simulink library "singleTether_cl"  (R2018b)
settings: Solver=VariableStepAuto  StartTime=0.0  StopTime=10.0  RelTol=1e-3
values from neighbouring files (symbols this model uses):
  ini_Ri_o = Ri_o    [singleTether_ts.m]
  ini_Vi_o = zeros(size(Vi_o))    [singleTether_ts.m]
  m_i = 2    [singleTether_ts.m]
  N = 20    [singleTether_ts.m]
libraries: tetherBuoyancyAndWeight_ul x1, tetherDragForce_ul x1, tetherInternalForces_ul x1
settings Model: Creator=asiddiq2  LastModifiedBy=asiddiq2

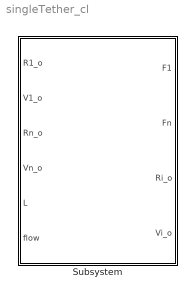
== system singleTether_cl ==
  Subsystem : Subsystem  mask{N=N, dia_t=0, E=0, rho_tether=0, Cd=0, zeta=0, rho_density=0, mass=0, ini_Rn_o=0, ini_R1_o=0}
      mask prompts: N "Number of nodes (N>=2)"; dia_t "Tether diameter (m)"; E "Tether youngs modulus (N/m^2)"; rho_tether "Tether density (kg/m^3)"; Cd "Tether drag coefficient"; zeta "Damping ratio"; rho_density "Fluid density"; mass "Vehicle mass"; ini_Rn_o "Initial vehicle attachment position vector"; ini_R1_o "Initial ground attachment position vector"
      mask DialogControl Container2 Prompt: Tether properties

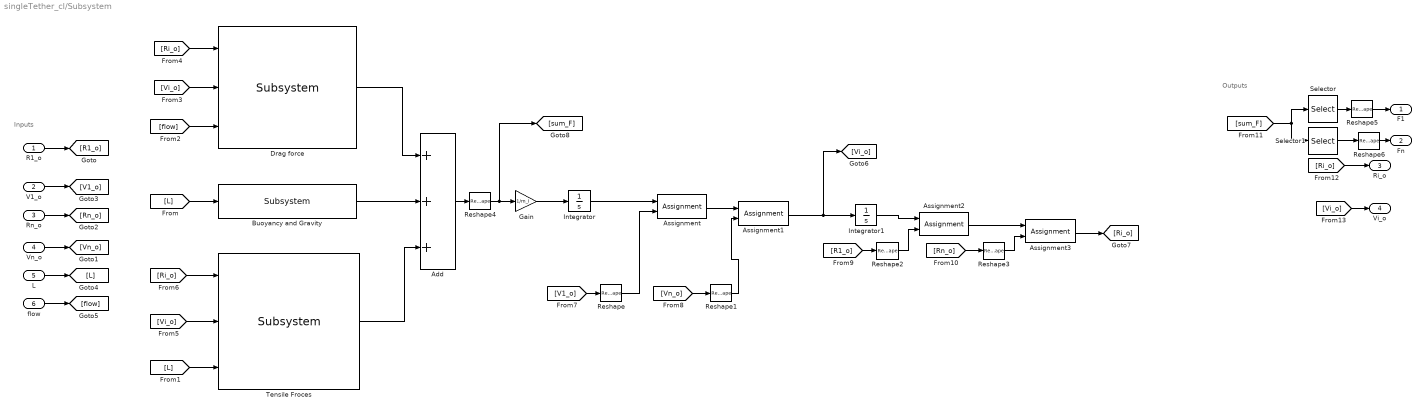
== system singleTether_cl/Subsystem ==
  note: Outputs
  note: Inputs
  R1_o : Inport
  V1_o : Inport  Port=2
  Rn_o : Inport  Port=3
  Vn_o : Inport  Port=4
  L : Inport  Port=5
  flow : Inport  Port=6
  Add : Sum  Inputs=+++
  Assignment : Assignment  NumberOfDimensions=2  DiagnosticForDimensions=Warning  IndexOptions=Index vector (dialog),Assign all  Indices=1,[1 2 3]  OutputSizes=1,1
  Assignment1 : Assignment  NumberOfDimensions=2  DiagnosticForDimensions=Warning  IndexOptions=Index vector (dialog),Assign all  Indices=N,[1 2 3]  OutputSizes=1,1
  Assignment2 : Assignment  NumberOfDimensions=2  DiagnosticForDimensions=Warning  IndexOptions=Index vector (dialog),Assign all  Indices=1,[1 2 3]  OutputSizes=1,1
  Assignment3 : Assignment  NumberOfDimensions=2  DiagnosticForDimensions=Warning  IndexOptions=Index vector (dialog),Assign all  Indices=N,[1 2 3]  OutputSizes=1,1
  Buoyancy and Gravity : tetherBuoyancyAndWeight_ul/Subsystem  N=N  dia_t=dia_t  rho_fluid=rho_fluid  rho_tether=rho_tether  g=9.81
  Drag force : tetherDragForce_ul/Subsystem  Cd=Cd  rho_fluid=rho_fluid  dia_t=dia_t
  Gain : Gain  Gain=1/m_i
  Integrator : Integrator  InitialCondition=ini_Vi_o
  Integrator1 : Integrator  InitialCondition=ini_Ri_o
  Reshape{,1..3} (4 alike) : Reshape  OutputDimensionality=Row vector (2-D)
  Reshape4 : Reshape  OutputDimensionality=Customize  OutputDimensions=[N,3]
  Reshape5 : Reshape  OutputDimensionality=Column vector (2-D)
  Reshape6 : Reshape  OutputDimensionality=Column vector (2-D)
  Selector : Selector  NumberOfDimensions=2  InputPortWidth=3  IndexOptions=Index vector (dialog),Select all  Indices=[1],1  OutputSizes=1,1
  Selector1 : Selector  NumberOfDimensions=2  InputPortWidth=3  IndexOptions=Index vector (dialog),Select all  Indices=[N],1  OutputSizes=1,1
  Tensile Froces : tetherInternalForces_ul/Subsystem  N=N  E=E  dia_t=dia_t  mass=mass  zeta=zeta
  F1 : Outport
  Fn : Outport  Port=2
  Ri_o : Outport  Port=3
  Vi_o : Outport  Port=4
  wires:
  R1_o/1 -> [R1_o]
  V1_o/1 -> [V1_o]
  Rn_o/1 -> [Rn_o]
  Vn_o/1 -> [Vn_o]
  L/1 -> [L]
  flow/1 -> [flow]
  [L] -> Buoyancy and Gravity/1
  [L] -> Tensile Froces/3
  [flow] -> Drag force/3
  Buoyancy and Gravity/1 -> Add/2
  Drag force/1 -> Add/1
  Tensile Froces/1 -> Add/3
  Gain/1 -> Integrator/1
  Integrator/1 -> Assignment/1
  [Vi_o] -> Drag force/2
  [Ri_o] -> Drag force/1
  [Vi_o] -> Tensile Froces/2
  [Ri_o] -> Tensile Froces/1
  [V1_o] -> Reshape/1
  Reshape/1 -> Assignment/2
  Assignment/1 -> Assignment1/1
  [Vn_o] -> Reshape1/1
  Reshape1/1 -> Assignment1/2
  Assignment1/1 -> [Vi_o], Integrator1/1
  [R1_o] -> Reshape2/1
  [Rn_o] -> Reshape3/1
  Reshape2/1 -> Assignment2/2
  Reshape3/1 -> Assignment3/2
  Integrator1/1 -> Assignment2/1
  Assignment2/1 -> Assignment3/1
  Assignment3/1 -> [Ri_o]
  Add/1 -> Reshape4/1
  [sum_F] -> Selector/1, Selector1/1
  [Ri_o] -> Ri_o/1
  [Vi_o] -> Vi_o/1
  Reshape4/1 -> [sum_F], Gain/1
  Selector1/1 -> Reshape6/1
  Reshape6/1 -> Fn/1
  Selector/1 -> Reshape5/1
  Reshape5/1 -> F1/1
